simulink model "main"  (R2021a)
settings: Solver=VariableStepAuto  StartTime=0.0  StopTime=1  RelTol=1e-3
settings Model: Creator=l.ribeiro-lustosa  LastModifiedBy=l.ribeiro-lustosa

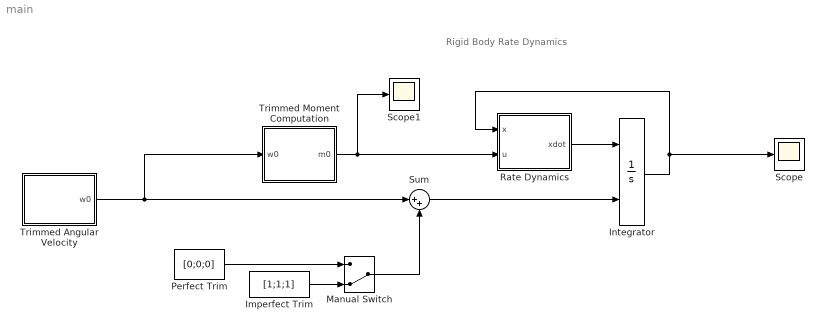
== system main ==
  note: Rigid Body Rate Dynamics
  Imperfect Trim : Constant  Value=[1;1;1]
  Integrator : Integrator  InitialConditionSource=external
  Manual Switch : ManualSwitch  CurrentSetting=0
  Perfect Trim : Constant  Value=[0;0;0]
  Rate Dynamics : MATLAB Function  TreatAsAtomicUnit=on
  Scope : Scope
  Scope1 : Scope
  Sum : Sum  Inputs=|++
  Trimmed Angular Velocity : MATLAB Function  TreatAsAtomicUnit=on
  Trimmed Moment Computation : MATLAB Function  TreatAsAtomicUnit=on
  wires:
  Rate Dynamics/1(xdot) -> Integrator/1
  Integrator/1 -> Scope/1, Rate Dynamics/1(x)
  Trimmed Angular Velocity/1(w0) -> Trimmed Moment Computation/1(w0), Sum/1
  Trimmed Moment Computation/1(m0) -> Scope1/1, Rate Dynamics/2(u)
  Sum/1 -> Integrator/2
  Perfect Trim/1 -> Manual Switch/1
  Imperfect Trim/1 -> Manual Switch/2
  Manual Switch/1 -> Sum/2

== matlab function main/Trimmed Moment Computation ==
  data: w0 input; m0 output; J parameter
function m0 = fcn(w0,J)

m0 = cross(w0,J*w0);

== matlab function main/Rate Dynamics ==
  data: x input; u input; xdot output; J parameter
function xdot = fcn(x,u,J)

%% Newton's Second Law for Rotation
xdot = J\( u - cross(x,J*x) );

== matlab function main/Trimmed Angular Velocity ==
  data: w0 output; J parameter
function w0 = fcn(J)

%% Eigenstructure information
[V,D] = eig(J);

%% Sorting eigenvalues in ascending order
[B,I] = sort(real([D(1,1);D(2,2);D(3,3)]));

%% Choosing a principal axes as desired trimmed condition
% Notice that choosing a principal axis will yield zero actuator moment for trim
% Choice of eigenvalues:
%   i=1 --> Least eigenvalue
%   i=2 --> Intermediate Axis
%   i=3 --> Largest eigenvalue
i=2;
w0 = 100*real(V(:,I(i)));
% You can also choose a random value, but that will require nonzero
% actuator moments!!
%w0 = 100*[1;2;3];
